simulink model "Test_Re_q_aero2_2dof"  (R2025a)
settings: Solver=ode1  StartTime=0.0  StopTime=90  FixedStep=0.002  RelTol=1e-3  EnableMultiTasking=on
values from neighbouring files (symbols this model uses):
  A = [0 0 -1.32553625076 2.23554898619e-20 0 0 0 0 1 0 -0.0857955963517 -4.06756404255e-26 ... (16 elements, 4x4)]    [PPlin.mat]    (also in aero2_2dof_ss_model.m = ss_d.A)
  B = [0  0; 0  0; 0.0231712909529  0.00988930486003; -0.0224305937979  0.0428923580462]    [PPlin.mat]    (also in aero2_2dof_ss_model.m = ss_d.B)
  C = [1  0  0  0; 0  1  0  0]    [PPlin.mat]    (also in aero2_2dof_ss_model.m = ss_d.C)
  D = [0  0; 0  0]    [PPlin.mat]    (also in aero2_2dof_ss_model.m = ss_d.D)
undefined symbols (not defined in the file or in its folder): HIL, qc_get_step_size
libraries: quarc_library x4
settings Model: SimulationMode=external  ExtModeTrigDuration=15000  Creator=MLevis  LastModifiedBy=khanh
settings SolverCC: AlgebraicLoopSolver=TrustRegion  PositivePriorityOrder=on
settings DataIOCC: LimitDataPoints=on  SaveFormat=Array  ReturnWorkspaceOutputs=off
settings DebuggingCC: SolverPrmCheckMsg=warning  UnconnectedInputMsg=warning  UnconnectedOutputMsg=warning  UnconnectedLineMsg=warning  SFUnexpectedBacktrackingDiag=warning  SFNoUnconditionalDefaultTransitionDiag=warning  SFExecutionAtInitializationDiag=none  ArithmeticOperatorsInVariantConditions=warning
settings ModelReferenceCC: EnableRefExpFcnMdlSchedulingChecks=on  PropagateSignalLabelsOutOfModel=off
settings SFSimCC: SimUseLocalCustomCode=off  CustomCodeUndefinedFunction=UseInterfaceOnly
settings RTWCC: SystemTargetFile=quarc_win64.tlc  TemplateMakefile=quarc_default_tmf  RTWUseLocalCustomCode=off  Toolchain=QUARC win64 | nmake (64-bit Windows)  BuildConfiguration=Faster Runs  GPUComputeCapability=3.5  DLArmComputeVersion=19.05  Description=QUARC Win64 Target Using Toolchain
settings CodeAppCC: StateflowObjectComments=on
settings STFCustomTargetCC: SystemTargetFile=quarc_win64.tlc  MultiwordLength=2048.0  DynamicStringBufferSize=256.0  ConcurrentExecutionCompliant=on  UseToolchainInfoCompliant=on
settings GRTTargetCC: ExtMode=on  ExtModeMexFile=quarc_comm  TargetLangStandard=C89/C90 (ANSI)  ParMdlRefBuildCompliant=off  CompOptLevelCompliant=off  CombineOutputUpdateFcns=off  MatFileLogging=off  CPPClassGenCompliant=off  GRTInterface=on
settings ConfigComp: CovMetricSettings=dw  CovSaveCumulativeToWorkspaceVar=on  CovSaveSingleToWorkspaceVar=on  CovExternalEMLEnable=off  CovSFcnEnable=off

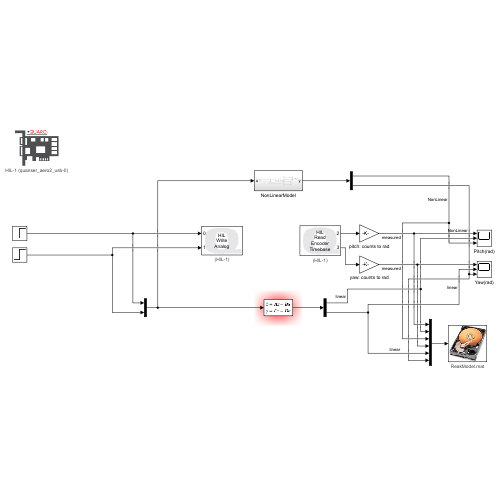
[thumbnail: Simulink's stored preview of the top-level diagram]
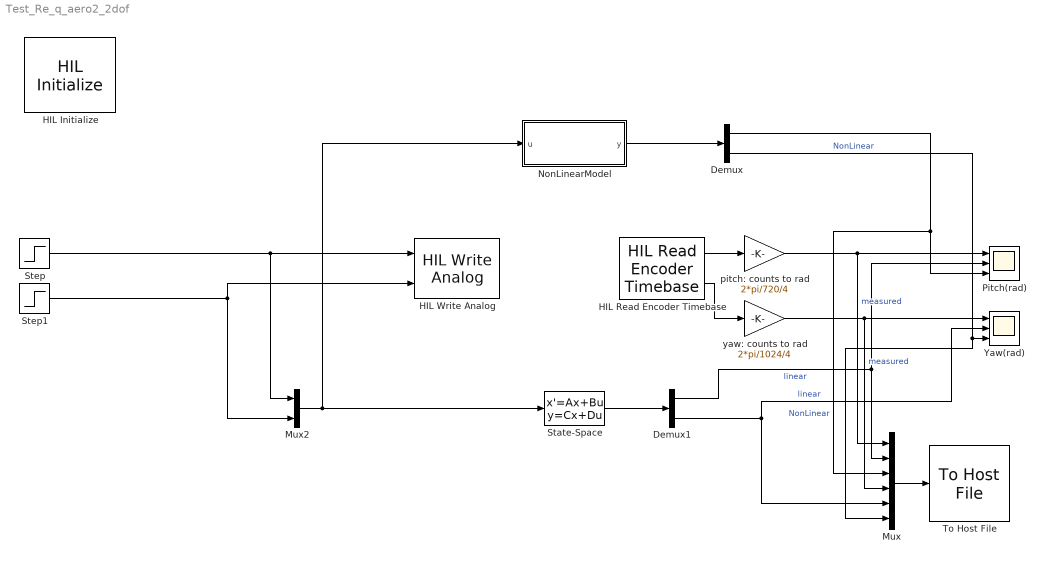
== system Test_Re_q_aero2_2dof ==
  Demux : Demux  Outputs=2
  Demux1 : Demux  Outputs=2
  HIL Initialize : quarc_library/Data Acquisition/Generic/Configuration/HIL Initialize  Priority=-99  object_name=HIL-1  board_type=quanser_aero2_usb  board_number=0  board_options=""  exclusive=off  active=off  hardware_clocks=[0]  clock_modes=[]  initial_clock_frequencies=[]  set_clock_params_at_start=off  set_clock_params_at_switch_in=off  set_clock_frequencies_at_start=off  set_clock_frequencies_at_switch_in=off  analog_input_channels=[0:1]  analog_input_configurations=[]  analog_input_maximums=3  analog_input_minimums=-3  set_analog_input_params_at_start=off  set_analog_input_params_at_switch_in=off  analog_output_channels=[0:1]  analog_output_maximums=24  analog_output_minimums=-24  initial_analog_outputs=[0]  final_analog_outputs=[0]  watchdog_analog_outputs=[0]  set_analog_output_params_at_start=off  set_analog_output_params_at_switch_in=off  set_analog_outputs_at_start=on  set_analog_outputs_at_switch_in=off  set_analog_outputs_at_terminate=on  set_analog_outputs_at_switch_out=off  set_analog_outputs_on_watchdog=on  digital_input_channels=[]  digital_output_channels=[0:1]  digital_output_configuration=[]  initial_digital_outputs=[1]  final_digital_outputs=[0]  watchdog_digital_outputs=[0]  set_digital_output_params_at_start=off  set_digital_output_params_at_switch_in=off  set_digital_outputs_at_start=on  set_digital_outputs_at_switch_in=off  set_digital_outputs_at_terminate=on  set_digital_outputs_at_switch_out=off  set_digital_outputs_on_watchdog=on  encoder_channels=[0:3]  quadrature=[4]  encoder_filter_frequency=[]  initial_encoder_counts=[0]  set_encoder_params_at_start=off  set_encoder_params_at_switch_in=off  set_encoder_counts_at_start=on  set_encoder_counts_at_switch_in=off  pwm_channels=[]  pwm_modes=[]  pwm_frequency=[]  pwm_configuration=[]  pwm_alignment=[]  pwm_polarity=[]  pwm_leading_deadband=[]  pwm_trailing_deadband=[]  initial_pwm_outputs=[]  final_pwm_outputs=[]  watchdog_pwm_outputs=[]  set_pwm_params_at_start=off  set_pwm_params_at_switch_in=off  set_pwm_outputs_at_start=off  set_pwm_outputs_at_switch_in=off  set_pwm_outputs_at_terminate=off  set_pwm_outputs_at_switch_out=off  set_pwm_outputs_on_watchdog=off  other_output_channels=[11000:11002]  initial_other_outputs=[0 1 0]  final_other_outputs=[1 0 0]  watchdog_other_outputs=[0 0 1]  set_other_outputs_at_start=on  set_other_outputs_at_switch_in=off  set_other_outputs_at_terminate=on  set_other_outputs_at_switch_out=off  set_other_outputs_on_watchdog=on
  HIL Read Encoder Timebase : quarc_library/Data Acquisition/Generic/Timebases/HIL Read Encoder Timebase  object_name=HIL-1  clock=0  channels=[2,3]  active=on  vector_output=off  data_type_mode=Inherit via back propagation  data_type=double  overflow_mode=Error on overflow  samples_in_buffer=max(ceil(1/qc_get_step_size), 1)
  HIL Write Analog : quarc_library/Data Acquisition/Generic/Immediate I//O/HIL Write Analog  object_name=HIL-1  channels=[0:1]  sample_time=-1  active=off  vector_input=off
  Mux : Mux  Inputs=6
  Mux2 : Mux  Inputs=2
  NonLinearModel : Subsystem
  Pitch(rad) : Scope  NumInputPorts=3
      settings: ActiveDisplayYMinimum=-2.2942881210344046  ActiveDisplayYMaximum=1.1978835120952036
  State-Space : StateSpace  A=A  B=B  C=C  D=D  InitialCondition=0
  Step : Step  After=5  SampleTime=0
  Step1 : Step  After=7  SampleTime=0
  To Host File : quarc_library/Sinks/To Host/To Host File  source=Specify via dialog (do not evaluate)  file_name=ReakModel.mat  variable_name=RealModel  decimation=1  sample_time=-1  file_format=MAT-file v.4  options=No header or footer  append=off  final_file_name=ReakModel.mat  encoding=Default  bitrate=0
  Yaw(rad) : Scope  NumInputPorts=3
      settings: ActiveDisplayYMinimum=110.72263842363324  ActiveDisplayYMaximum=118.81851737273804  DataLoggingVariableName=ScopeData3
  pitch: counts to rad : Gain  Gain=2*pi/720/4
  yaw: counts to rad : Gain  Gain=2*pi/1024/4
  wires:
  HIL Read Encoder Timebase/2 -> yaw: counts to rad/1
  HIL Read Encoder Timebase/1 -> pitch: counts to rad/1
  Step/1 -> HIL Write Analog/1, Mux2/1
  Mux2/1 -> State-Space/1, NonLinearModel/1(u)
  Step1/1 -> Mux2/2, HIL Write Analog/2
  pitch: counts to rad/1 -> Mux/1, Pitch(rad)/1  "measured"
  yaw: counts to rad/1 -> Mux/4, Yaw(rad)/1  "measured"
  Demux1/1 -> Pitch(rad)/2, Mux/2  "linear"
  Demux1/2 -> Mux/5, Yaw(rad)/2  "linear"
  Mux/1 -> To Host File/1
  State-Space/1 -> Demux1/1
  NonLinearModel/1(y) -> Demux/1
  Demux/1 -> Mux/3, Pitch(rad)/3  "NonLinear"
  Demux/2 -> Mux/6, Yaw(rad)/3  "NonLinear"

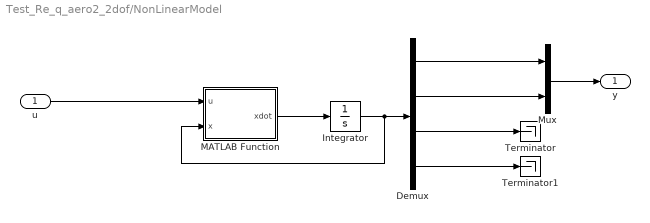
== system Test_Re_q_aero2_2dof/NonLinearModel ==
  u : Inport  PortDimensions=2
  Demux : Demux
  Integrator : Integrator  InitialCondition=zeros(4,1)
  MATLAB Function : MATLAB Function  TreatAsAtomicUnit=on
  Mux : Mux  Inputs=2
  Terminator : Terminator
  Terminator1 : Terminator
  y : Outport
  wires:
  Mux/1 -> y/1
  MATLAB Function/1(xdot) -> Integrator/1
  Integrator/1 -> MATLAB Function/2(x), Demux/1
  Demux/2 -> Mux/2
  Demux/4 -> Terminator1/1
  u/1 -> MATLAB Function/1(u)
  Demux/1 -> Mux/1
  Demux/3 -> Terminator/1

== matlab function Test_Re_q_aero2_2dof/NonLinearModel/MATLAB Function ==
  data: u input size=2; xdot output size=4; x input size=4
function xdot  = fcn(u, x)

theta = x(1);
psi = x(2);
theta_dot = x(3);
psi_dot = x(4);

Vp = u(1);
Vy = u(2);

% Parameters
% distance from pivot to center of rotor/propeller (m)
Dt = 0.16743; 
% total aero body mass (kg)
Mb = 1.07; 
% distance from aero body plane to center of mass below (m)
l = 2.4e-3; 
% Moment of inertia about pitch-axis (kg-m^2)
Jp = 23188500.45 / 1000 * 0.001^2; % from CAD: 23188500.45 g-mm^2
% Moment of inertia about pitch-axis (kg-m^2)
Jy = 23810415.95 / 1000 * 0.001^2; % from CAD: 23810415.95 g-mm^2;
% Gravity (m/s^2)
g = 9.81;
% Stiffness (N-m/V)
Ksp = 0.00744;
% Damping (N-m/V)
Dp = 0.00199;
% Pitch thrust gain (N/V)
Kpp = 0.00321;
% Pitch from yaw thrust gain (N/V)
Kpy = 0.00137;
% Damping (N-m/V)
Dy = 0.00192;
% Thrust (N-m/V)
Kyy = 0.00610;
% Yaw from pitch thrust gain (N/V)
Kyp = -0.00319;

theta_ddot = (Dt*Kpp*Vp + ...
              Dt*Kpy*Vy - ...
              Mb*g*l*cos(theta) - ...
              Dp*theta_dot - ...
              Ksp*theta - ...
              Mb*psi_dot^2*l^2*sin(theta)*cos(theta)) / (Jp + Mb*l^2);
psi_ddot = (Dt*Kyp*Vp + ...
            Kyy*Vy - ...
            Dy*psi_dot + ...
            Mb*l^2*psi_dot*theta_dot*sin(2*theta)) / (Jy + Mb*l^2*cos(theta)^2);

xdot = [theta_dot, psi_dot, theta_ddot, psi_ddot]';
